simulink library "Copy_of_GFe_Lib"  (R2018b)
settings: Solver=VariableStepAuto  StartTime=0.0  StopTime=10.0  RelTol=1e-3
undefined symbols (not defined in the file or in its folder): fb, Ib2, Ki_i, Kp_i, Lf_pu, Sb, Solver_Time_Step, Time_Step, Va0, Vb0, Vb1, Vb2, Vc0, Vm0_d, Vm0_q, Vvsc0, wb, Zb
libraries: powerlib x20, Control_Lib x8, simulink x6
(part 1 of 2)
settings Model: Creator=Frederic_Colas  LastModifiedBy=Frederic_Colas
settings SFSimCC: SimUseLocalCustomCode=off
settings RTWCC: RTWUseLocalCustomCode=off

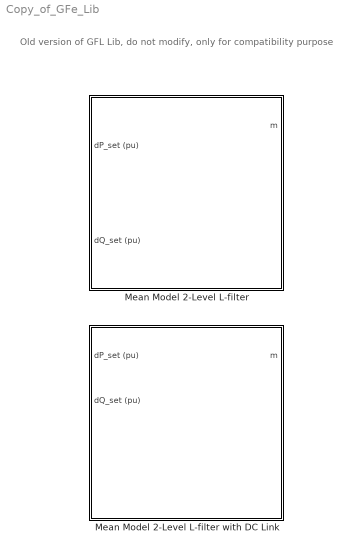
== system Copy_of_GFe_Lib ==
  note: Old version of GFL Lib, do not modify, only for compatibility purpose
  Mean Model 2-Level L-filter : Subsystem  mask(VSC){fn=50.0, Sn=1e9, Pn=1e9, Udcn=640e3, Time_Step=Time_Step, Un1=320e3, Un2=400e3, m=1, Rt_pu=0.005, Lt_pu=0.15, Lm_pu=inf, Rm_pu=inf, Tr_PLL=100, wn_i=1500, zeta_i=0.7, Kffi=on, Filtre_FF=on, w_ff=1000, QV=Reactive Power Control, w_P=10, w_V=50, w_LPF=4000, Imax=5, Iqmax=5, K_FRT=0, LFpopup=PQ, P0=0, Q0=0, V0=1.0108, Theta0=0.4912}
      mask prompts: fn "Nominal Frequency (Hz)"; Sn "Nominal Apparent Power (VA)"; Pn "Nominal Power (W)"; Udcn "Nominal DC Voltage (V)"; Time_Step "Sample Time (s)"; Un1 "VSC side Nominal Ph-Ph Voltage (V)"; Un2 "Grid side Nominal Ph-Ph Voltage (V)"; m "Transformer's ratio (p.u)"; Rt_pu "R (pu)"; Lt_pu "L (pu)"; Lm_pu "Rm (pu)"; Rm_pu "Lm (pu)"; Tr_PLL "Time response (ms)"; wn_i "Bandwidth (rad/s)"; zeta_i "Damping factor"; Kffi "Feedfoward Enable"; Filtre_FF "Filter of ff enable"; w_ff "Cutoff frequency (rad/s)"; QV "Mode"; w_P "Power control bandwidth"; w_V "Voltage control bandwidth"; w_LPF "Low-pass filters bandwidth"; Imax "Maximum current"; Iqmax "Maximum quadrature current"; K_FRT "LVRT block enabled (1) or disabled (0)"; P0 "Initial Active Power (pu)"; Q0 "Initial Reactive Power (pu)"; V0 "Initial Voltage (pu)"; Theta0 "Initial Angle (°)"
      mask init:
      | Init_Base;
      | Init_LF_L;
      | Init_GFL;
      settings: OpenFcn=|
      | NameStr = get_param(gcb,'Name');
      | open_system(gcbh, 'Mask');
      | 
      | h2AllOpenDlgs = DAStudio.ToolRoot.getOpenDialogs;
      | 
      | for i=1:length(h2AllOpenDlgs)
      |     try
      |          %disp(h2AllOpenDlgs(i).getSource.getBlock.Name);
      |         Dialog_block_name = h2AllOpenDlgs(i).getSource.getBlock.Name;
      |          %strcmp(Dialog_block_name, NameStr),
      |         if (strcmp(h2AllOpenDlgs(i).getSource.getBlock.Name, NameStr))
      |             iPos = h2AllOpenDlgs(i).position;
      |             h2AllOpenDlgs(i).position = [iPos(1)   iPos(2)   iPos(3)*1.4   iPos(4)];
      |         end
      |     end
      | end
      mask TypeOptions QV: Voltage Control | Reactive Power Control
      mask TypeOptions LFpopup: Swing | PQ | PV
      mask Callback LFpopup:
      | % Get the mask parameter values. This is a cell
      | %   array of character vectors.
      | maskStr = get_param(gcb,'LFpopup');
      | p=Simulink.Mask.get(gcb);
      | 
      | % The pop-up menu is the first mask parameter.
      | %   Check the value selected in the pop-up
      | if strcmp(maskStr,'Swing'),
      | 
      |     % Set the visibility of both parameters on when
      |     %   User-defined is selected in the pop-up.
      |     p.getParameter('P0').Visible='off';
      |     p.getParameter('Q0').Visible='off';
      |     p.getParameter('V0').Visible='on';
      |     p.getParameter('Theta0').Visible='on';
      |     set_param([gcb '/Source_For_LF'],'BusType','swing');
      | 
      | elseif strcmp(maskStr,'PQ'),
      | 
      |     % Set the visibility of both parameters on when
      |     %   User-defined is selected in the pop-up.
      |     p.getParameter('P0').Visible='on';
      |     p.getParameter('Q0').Visible='on';
      |     p.getParameter('V0').Visible='off';
      |     p.getParameter('Theta0').Visible='off';
      |     set_param([gcb '/Source_For_LF'],'BusType','PQ');
      | 
      |     % Turn off the visibility of the Value field
      |     %   when User-defined is not selected.
      | else
      | 
      |     % Set the visibility of both parameters on when
      |     %   User-defined is selected in the pop-up.
      |     p.getParameter('P0').Visible='on';
      |     p.getParameter('Q0').Visible='off';
      |     p.getParameter('V0').Visible='on';
      |     p.getParameter('Theta0').Visible='off';
      |     set_param([gcb '/Source_For_LF'],'BusType','PV');
      | 
      | end
      mask DialogControl Nominal_Param Prompt: Nominal Value
      mask DialogControl Container20 Prompt: Output Transformer
      mask DialogControl Control_Param Prompt: Control Parameter
      mask DialogControl Container13 Prompt: PLL
      mask DialogControl Container14 Prompt: Current Loop
      mask DialogControl Container11 Prompt: Outer loop
      mask DialogControl Container15 Prompt: Control gains
      mask DialogControl Container16 Prompt: Current saturations
      mask DialogControl Container21 Prompt: LVRT
      mask DialogControl LF_Param Prompt: Loadflow
      mask DialogControl Control4 Prompt: Initial Operating Point
      mask DialogControl Container24 Prompt: VSC side
      mask DialogControl LF_vsc_str Prompt: V0 = 1.0108 pu, Angle = 0.4912°
      mask DialogControl Container25 Prompt: PCC
      mask DialogControl LF_pcc_str Prompt: V0 = 1.0108 pu, Angle = 0.4912°
      mask DialogControl LF_pcc_Power_str Prompt: P0 = 0 pu, Q0 = 0 pu
      mask DialogControl UpdateLoadflow Prompt: Update Loadflow
      mask DialogControl UpdateLoadflow Callback: LoadFlow_VSC
      mask Display:
      | x1=0.05;
      | y1=0.2;
      | %
      | plot([0.5 0.5]+x1,[0.97,0.8]-y1)
      | plot([0.5 0.32]+x1,[0.80 0.71]-y1)
      | plot([0.32 0.32]+x1,[0.80 0.52]-y1)
      | plot([0.32 0.5]+x1,[0.62 0.52]-y1)
      | plot([0.5 0.5]+x1,[0.52 0.35]-y1)
      | plot([0.45 0.5 0.43]+x1,[0.59 0.52 0.51]-y1)
      | %
      | plot([0.28 0.28]+x1,[0.74 0.58]-y1)
      | plot([0.28 0.20]+x1,[0.66 0.66]-y1)
      | %
      | plot([0.5 0.63]+x1,[0.84 0.84]-y1)
      | plot([0.63 0.63]+x1,[0.84 0.72]-y1)
      | plot([0.63 0.59]+x1,[0.72 0.65]-y1)
      | plot([0.63 0.67]+x1,[0.72 0.65]-y1)
      | plot([0.59 0.67]+x1,[0.65 0.65]-y1)
      | plot([0.63 0.63]+x1,[0.65 0.47]-y1)
      | plot([0.5 0.63]+x1,[0.47 0.47]-y1)
      | plot([0.58 0.67]+x1,[0.72 0.72]-y1)
      | %
      | color('blue')
      | text(0.3,0.10,'L-Filter GFL')
      | 
      | port_label('input',1,'\DeltaP (pu)','texmode','on');
      | port_label('input',2,'\DeltaQ (pu)','texmode','on');
      | port_label('output',1,'m');
      | port_label('rconn',1,'A');
      | port_label('rconn',2,'B');
      | port_label('rconn',3,'C');
  Mean Model 2-Level L-filter with DC Link : Subsystem  mask(VSC){fn=50.0, Sn=1e9, Pn=1e9, Udcn=640e3, Time_Step=Time_Step, Un1=320e3, Un2=400e3, m=1, Rt_pu=0.005, Lt_pu=0.15, Lm_pu=inf, Rm_pu=inf, H_DC=40, Tr_PLL=100, wn_i=1500, zeta_i=0.7, Kffi=on, Filtre_FF=on, w_ff=1000, QV=Reactive Power Control, w_P=10, w_V=50, w_LPF=4000, Imax=5, Iqmax=5, K_FRT=0, LFpopup=PQ, P0=0, Q0=0, V0=1.0108, Theta0=0.4912}
      mask prompts: fn "Nominal Frequency (Hz)"; Sn "Nominal Apparent Power (VA)"; Pn "Nominal Power (W)"; Udcn "Nominal DC Voltage (V)"; Time_Step "Sample Time (s)"; Un1 "VSC side Nominal Ph-Ph Voltage (V)"; Un2 "Grid side Nominal Ph-Ph Voltage (V)"; m "Transformer's ratio (p.u)"; Rt_pu "R (pu)"; Lt_pu "L (pu)"; Lm_pu "Rm (pu)"; Rm_pu "Lm (pu)"; H_DC "DC inertias (ms)"; Tr_PLL "Time response (ms)"; wn_i "Bandwidth (rad/s)"; zeta_i "Damping factor"; Kffi "Feedfoward Enable"; Filtre_FF "Filter of ff enable"; w_ff "Cutoff frequency (rad/s)"; QV "Mode"; w_P "Power control bandwidth"; w_V "Voltage control bandwidth"; w_LPF "Low-pass filters bandwidth"; Imax "Maximum current"; Iqmax "Maximum quadrature current"; K_FRT "LVRT block enabled (1) or disabled (0)"; P0 "Initial Active Power (pu)"; Q0 "Initial Reactive Power (pu)"; V0 "Initial Voltage (pu)"; Theta0 "Initial Angle (°)"
      mask init:
      | Init_Base;
      | Init_LF_L;
      | Init_GFL;
      | Init_Cdc;
      settings: OpenFcn=|
      | NameStr = get_param(gcb,'Name');
      | open_system(gcbh, 'Mask');
      | 
      | h2AllOpenDlgs = DAStudio.ToolRoot.getOpenDialogs;
      | 
      | for i=1:length(h2AllOpenDlgs)
      |     try
      |          %disp(h2AllOpenDlgs(i).getSource.getBlock.Name);
      |         Dialog_block_name = h2AllOpenDlgs(i).getSource.getBlock.Name;
      |          %strcmp(Dialog_block_name, NameStr),
      |         if (strcmp(h2AllOpenDlgs(i).getSource.getBlock.Name, NameStr))
      |             iPos = h2AllOpenDlgs(i).position;
      |             h2AllOpenDlgs(i).position = [iPos(1)   iPos(2)   iPos(3)*1.4   iPos(4)];
      |         end
      |     end
      | end
      mask TypeOptions QV: Voltage Control | Reactive Power Control
      mask TypeOptions LFpopup: Swing | PQ | PV
      mask Callback LFpopup:
      | % Get the mask parameter values. This is a cell
      | %   array of character vectors.
      | maskStr = get_param(gcb,'LFpopup');
      | p=Simulink.Mask.get(gcb);
      | 
      | % The pop-up menu is the first mask parameter.
      | %   Check the value selected in the pop-up
      | if strcmp(maskStr,'Swing'),
      | 
      |     % Set the visibility of both parameters on when
      |     %   User-defined is selected in the pop-up.
      |     p.getParameter('P0').Visible='off';
      |     p.getParameter('Q0').Visible='off';
      |     p.getParameter('V0').Visible='on';
      |     p.getParameter('Theta0').Visible='on';
      |     set_param([gcb '/Source_For_LF'],'BusType','swing');
      | 
      | elseif strcmp(maskStr,'PQ'),
      | 
      |     % Set the visibility of both parameters on when
      |     %   User-defined is selected in the pop-up.
      |     p.getParameter('P0').Visible='on';
      |     p.getParameter('Q0').Visible='on';
      |     p.getParameter('V0').Visible='off';
      |     p.getParameter('Theta0').Visible='off';
      |     set_param([gcb '/Source_For_LF'],'BusType','PQ');
      | 
      |     % Turn off the visibility of the Value field
      |     %   when User-defined is not selected.
      | else
      | 
      |     % Set the visibility of both parameters on when
      |     %   User-defined is selected in the pop-up.
      |     p.getParameter('P0').Visible='on';
      |     p.getParameter('Q0').Visible='off';
      |     p.getParameter('V0').Visible='on';
      |     p.getParameter('Theta0').Visible='off';
      |     set_param([gcb '/Source_For_LF'],'BusType','PV');
      | 
      | end
      mask DialogControl Nominal_Param Prompt: Nominal Value
      mask DialogControl Container20 Prompt: Passive Components
      mask DialogControl Container29 Prompt: Output Transformer
      mask DialogControl Container28 Prompt: DC Link
      mask DialogControl Control_Param Prompt: Control Parameter
      mask DialogControl Container13 Prompt: PLL
      mask DialogControl Container14 Prompt: Current Loop
      mask DialogControl Container11 Prompt: Outer loop
      mask DialogControl Container15 Prompt: Control gains
      mask DialogControl Container16 Prompt: Current saturations
      mask DialogControl Container21 Prompt: LVRT
      mask DialogControl LF_Param Prompt: Loadflow
      mask DialogControl Control4 Prompt: Initial Operating Point
      mask DialogControl Container24 Prompt: VSC side
      mask DialogControl LF_vsc_str Prompt: V0 = 1.0108 pu, Angle = 0.4912°
      mask DialogControl Container25 Prompt: PCC
      mask DialogControl LF_pcc_str Prompt: V0 = 1.0108 pu, Angle = 0.4912°
      mask DialogControl LF_pcc_Power_str Prompt: P0 = 0 pu, Q0 = 0 pu
      mask DialogControl UpdateLoadflow Prompt: Update Loadflow
      mask DialogControl UpdateLoadflow Callback: LoadFlow_VSC
      mask Display:
      | x1=0.05;
      | y1=0.2;
      | %
      | plot([0.5 0.5]+x1,[0.97,0.8]-y1)
      | plot([0.5 0.32]+x1,[0.80 0.71]-y1)
      | plot([0.32 0.32]+x1,[0.80 0.52]-y1)
      | plot([0.32 0.5]+x1,[0.62 0.52]-y1)
      | plot([0.5 0.5]+x1,[0.52 0.35]-y1)
      | plot([0.45 0.5 0.43]+x1,[0.59 0.52 0.51]-y1)
      | %
      | plot([0.28 0.28]+x1,[0.74 0.58]-y1)
      | plot([0.28 0.20]+x1,[0.66 0.66]-y1)
      | %
      | plot([0.5 0.63]+x1,[0.84 0.84]-y1)
      | plot([0.63 0.63]+x1,[0.84 0.72]-y1)
      | plot([0.63 0.59]+x1,[0.72 0.65]-y1)
      | plot([0.63 0.67]+x1,[0.72 0.65]-y1)
      | plot([0.59 0.67]+x1,[0.65 0.65]-y1)
      | plot([0.63 0.63]+x1,[0.65 0.47]-y1)
      | plot([0.5 0.63]+x1,[0.47 0.47]-y1)
      | plot([0.58 0.67]+x1,[0.72 0.72]-y1)
      | %
      | color('blue')
      | text(0.3,0.10,'L-Filter GFL')
      | 
      | port_label('input',1,'\DeltaP (pu)','texmode','on');
      | port_label('input',2,'\DeltaQ (pu)','texmode','on');
      | port_label('output',1,'m');
      | port_label('rconn',1,'A');
      | port_label('rconn',2,'B');
      | port_label('rconn',3,'C');
      | port_label('lconn',1,'+');
      | port_label('lconn',2,'-');

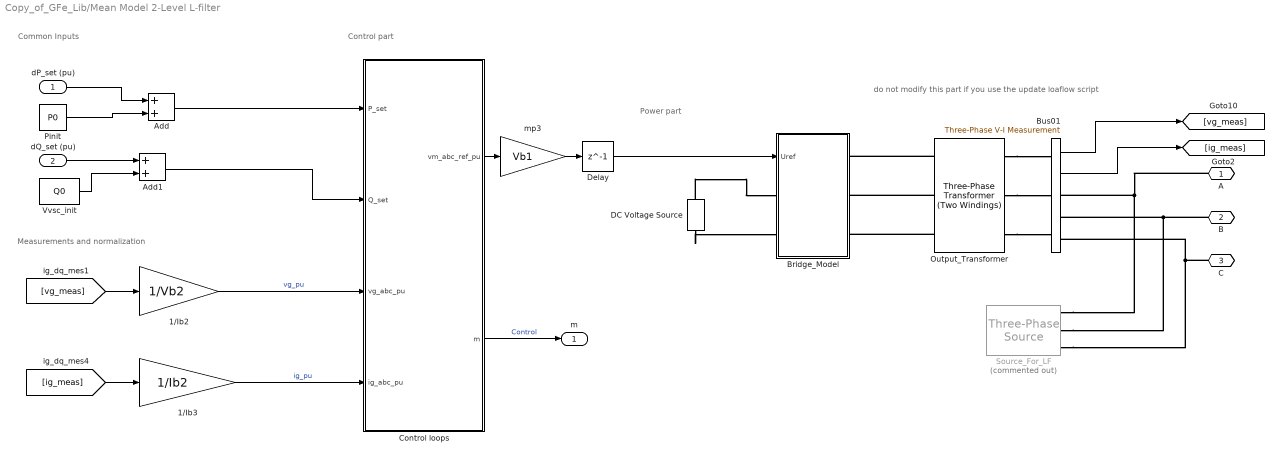
== system Copy_of_GFe_Lib/Mean Model 2-Level L-filter ==
  note: Control part
  note: Measurements and normalization
  note: Power part
  note: Common Inputs
  note: do not modify this part if you use the update loaflow script
  dP_set (pu) : Inport
  dQ_set (pu) : Inport  Port=2
  1/Ib2 : Gain  Gain=1/Vb2
  1/Ib3 : Gain  Gain=1/Ib2
  Add : Sum
  Add1 : Sum
  Bridge_Model : Subsystem
  Bus01 : powerlib/Measurements/Three-Phase V-I Measurement  VoltageMeasurement=phase-to-ground  SetLabelV=off  LabelV=Vabc  Vpu=off  VpuLL=off  CurrentMeasurement=yes  SetLabelI=off  LabelI=Iabc  Ipu=off  Pbase=100e6  Vbase=500e3  OutputType=Complex  PhasorSimulation=off  PSBequivalent=0
  Control loops : Subsystem
  DC Voltage Source : powerlib/Electrical Sources/DC Voltage Source  Amplitude=Udcn  Measurements=Voltage
  Delay : Delay  DelayLength=1  InitialCondition=[Va0 Vb0 Vc0]  SampleTime=Solver_Time_Step
  Output_Transformer : powerlib/Elements/Three-Phase Transformer (Two Windings)  Winding1Connection=Yg  Winding2Connection=Yg  CoreType=Three single-phase transformers  SetSaturation=off  Hysteresis=off  DataFile='hysteresis'  SetInitialFlux=off  Measurements=None  UNITS=pu  NominalPower=[Sn , fb]  Winding1=[Un1 , Rt_pu/2*(m^2), Lt_pu/2*(m^2)]  Winding2="[Un2*m ,  Rt_pu/2*(m^2), Lt_pu/2*(m^2)]"  Rm=Rm_pu  Lm=Lm_pu  L0=0.5  Saturation=[ 0,0 ; 0.0024,1.2 ; 1.0,1.52 ]  InitialFluxes=[ 0.8 , -0.8 , 0.7 ]  BreakLoop=off  DiscreteSolver=Trapezoidal iterative  DataType=off  TransfoNumber=1
  Pinit : Constant  Value=P0
  Source_For_LF : powerlib/Electrical Sources/Three-Phase Source  Commented=on  InternalConnection=Yg  VoltagePhases=off  Voltage=(400000)*1.01081  PhaseAngle=0.4912  Voltage_phases=[25e3 25e3 25e3]/sqrt(3)  PhaseAngles_phases=[0 -120 +120]  Frequency=fb  NonIdealSource=off  SpecifyImpedance=off  Resistance=0  Inductance=0  ShortCircuitLevel=100e6  BaseVoltage=Un  XRratio=7  BusType=PQ  Pref=P0*Sb  Qref=Q0*Sb  Prefabc=[10e3, 10e3, 10e3]  Qrefabc=[0, 0, 0]  Qmin=-inf  Qmax=inf
  Vvsc_init : Constant  Value=Q0
  mp3 : Gain  Gain=Vb1
  A : PMIOPort  Side=Right
  B : PMIOPort  Port=2  Side=Right
  C : PMIOPort  Port=3  Side=Right
  m : Outport  VectorParamsAs1DForOutWhenUnconnected=off
  wires:
  [ig_meas] -> 1/Ib3/1
  dQ_set (pu)/1 -> Add1/1
  Vvsc_init/1 -> Add1/2
  Pinit/1 -> Add/2
  dP_set (pu)/1 -> Add/1
  Add1/1 -> Control loops/2(Q_set)
  Control loops/1(vm_abc_ref_pu) -> mp3/1
  [vg_meas] -> 1/Ib2/1
  1/Ib2/1 -> Control loops/3(vg_abc_pu)  "vg_pu"
  1/Ib3/1 -> Control loops/4(ig_abc_pu)  "ig_pu"
  mp3/1 -> Delay/1
  Control loops/2(m) -> m/1  "Control"
  Add/1 -> Control loops/1(P_set)
  Bus01/1 -> [vg_meas]
  Delay/1 -> Bridge_Model/1(Uref)
  Bus01/2 -> [ig_meas]
  connections:
  B/RConn1 -- Source_For_LF/RConn2 -- Bus01/RConn2
  C/RConn1 -- Source_For_LF/RConn3 -- Bus01/RConn3
  A/RConn1 -- Source_For_LF/RConn1 -- Bus01/RConn1
  DC Voltage Source/RConn1 -- Bridge_Model/LConn1
  Output_Transformer/LConn3 -- Bridge_Model/RConn3
  Output_Transformer/LConn1 -- Bridge_Model/RConn1
  DC Voltage Source/LConn1 -- Bridge_Model/LConn2
  Output_Transformer/RConn2 -- Bus01/LConn2
  Output_Transformer/RConn1 -- Bus01/LConn1
  Output_Transformer/LConn2 -- Bridge_Model/RConn2
  Output_Transformer/RConn3 -- Bus01/LConn3

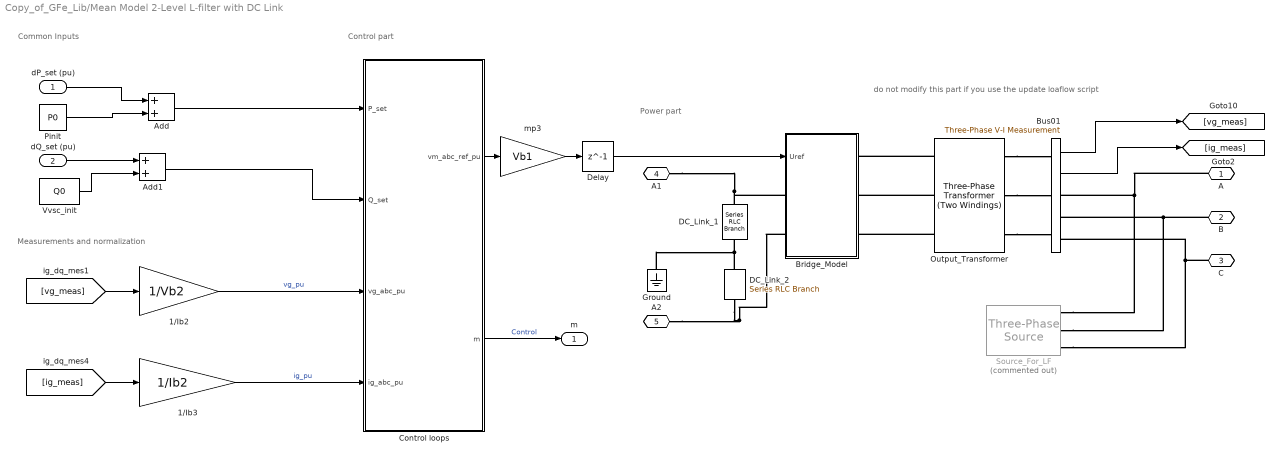
== system Copy_of_GFe_Lib/Mean Model 2-Level L-filter with DC Link ==
  note: Control part
  note: Measurements and normalization
  note: Power part
  note: Common Inputs
  note: do not modify this part if you use the update loaflow script
  dP_set (pu) : Inport
  dQ_set (pu) : Inport  Port=2
  1/Ib2 : Gain  Gain=1/Vb2
  1/Ib3 : Gain  Gain=1/Ib2
  Add : Sum
  Add1 : Sum
  Bridge_Model : Subsystem
  Bus01 : powerlib/Measurements/Three-Phase V-I Measurement  VoltageMeasurement=phase-to-ground  SetLabelV=off  LabelV=Vabc  Vpu=off  VpuLL=off  CurrentMeasurement=yes  SetLabelI=off  LabelI=Iabc  Ipu=off  Pbase=100e6  Vbase=500e3  OutputType=Complex  PhasorSimulation=off  PSBequivalent=0
  Control loops : Subsystem
  DC_Link_1 : powerlib/Elements/Series RLC Branch  LConnTagsString=__new0  RConnTagsString=__new0  BranchType=C  Resistance=1  Inductance=1e-3  SetiL0=off  InitialCurrent=0  Capacitance=0.00039063  Setx0=on  InitialVoltage=Udcn/2  Measurements=None
  DC_Link_2 : powerlib/Elements/Series RLC Branch  LConnTagsString=__new0  RConnTagsString=__new0  BranchType=C  Resistance=1  Inductance=1e-3  SetiL0=off  InitialCurrent=0  Capacitance=0.00039063  Setx0=on  InitialVoltage=Udcn/2  Measurements=None
  Delay : Delay  DelayLength=1  InitialCondition=[Va0 Vb0 Vc0]  SampleTime=Solver_Time_Step
  Ground : powerlib/Elements/Ground  LConnTagsString=a
  Output_Transformer : powerlib/Elements/Three-Phase Transformer (Two Windings)  Winding1Connection=Yg  Winding2Connection=Yg  CoreType=Three single-phase transformers  SetSaturation=off  Hysteresis=off  DataFile='hysteresis'  SetInitialFlux=off  Measurements=None  UNITS=pu  NominalPower=[Sn , fb]  Winding1=[Un1 , Rt_pu/2*(m^2), Lt_pu/2*(m^2)]  Winding2="[Un2*m ,  Rt_pu/2*(m^2), Lt_pu/2*(m^2)]"  Rm=Rm_pu  Lm=Lm_pu  L0=0.5  Saturation=[ 0,0 ; 0.0024,1.2 ; 1.0,1.52 ]  InitialFluxes=[ 0.8 , -0.8 , 0.7 ]  BreakLoop=off  DiscreteSolver=Trapezoidal iterative  DataType=off  TransfoNumber=1
  Pinit : Constant  Value=P0
  Source_For_LF : powerlib/Electrical Sources/Three-Phase Source  Commented=on  InternalConnection=Yg  VoltagePhases=off  Voltage=(400000)*1.01081  PhaseAngle=0.4912  Voltage_phases=[25e3 25e3 25e3]/sqrt(3)  PhaseAngles_phases=[0 -120 +120]  Frequency=fb  NonIdealSource=off  SpecifyImpedance=off  Resistance=0  Inductance=0  ShortCircuitLevel=100e6  BaseVoltage=Un  XRratio=7  BusType=PQ  Pref=P0*Sb  Qref=Q0*Sb  Prefabc=[10e3, 10e3, 10e3]  Qrefabc=[0, 0, 0]  Qmin=-inf  Qmax=inf
  Vvsc_init : Constant  Value=Q0
  mp3 : Gain  Gain=Vb1
  A : PMIOPort  Side=Right
  B : PMIOPort  Port=2  Side=Right
  C : PMIOPort  Port=3  Side=Right
  A1 : PMIOPort  Port=4  Side=Left
  A2 : PMIOPort  Port=5  Side=Left
  m : Outport  VectorParamsAs1DForOutWhenUnconnected=off
  wires:
  [ig_meas] -> 1/Ib3/1
  dQ_set (pu)/1 -> Add1/1
  Vvsc_init/1 -> Add1/2
  Pinit/1 -> Add/2
  dP_set (pu)/1 -> Add/1
  Add1/1 -> Control loops/2(Q_set)
  Control loops/1(vm_abc_ref_pu) -> mp3/1
  [vg_meas] -> 1/Ib2/1
  1/Ib2/1 -> Control loops/3(vg_abc_pu)  "vg_pu"
  1/Ib3/1 -> Control loops/4(ig_abc_pu)  "ig_pu"
  mp3/1 -> Delay/1
  Control loops/2(m) -> m/1  "Control"
  Add/1 -> Control loops/1(P_set)
  Bus01/1 -> [vg_meas]
  Delay/1 -> Bridge_Model/1(Uref)
  Bus01/2 -> [ig_meas]
  connections:
  B/RConn1 -- Source_For_LF/RConn2 -- Bus01/RConn2
  C/RConn1 -- Source_For_LF/RConn3 -- Bus01/RConn3
  A/RConn1 -- Source_For_LF/RConn1 -- Bus01/RConn1
  Output_Transformer/LConn3 -- Bridge_Model/RConn3
  Output_Transformer/LConn1 -- Bridge_Model/RConn1
  Output_Transformer/RConn2 -- Bus01/LConn2
  Output_Transformer/RConn1 -- Bus01/LConn1
  Output_Transformer/LConn2 -- Bridge_Model/RConn2
  Output_Transformer/RConn3 -- Bus01/LConn3
  DC_Link_1/LConn1 -- A1/RConn1 -- Bridge_Model/LConn1
  DC_Link_2/RConn1 -- Bridge_Model/LConn2 -- A2/RConn1
  DC_Link_1/RConn1 -- DC_Link_2/LConn1 -- Ground/LConn1

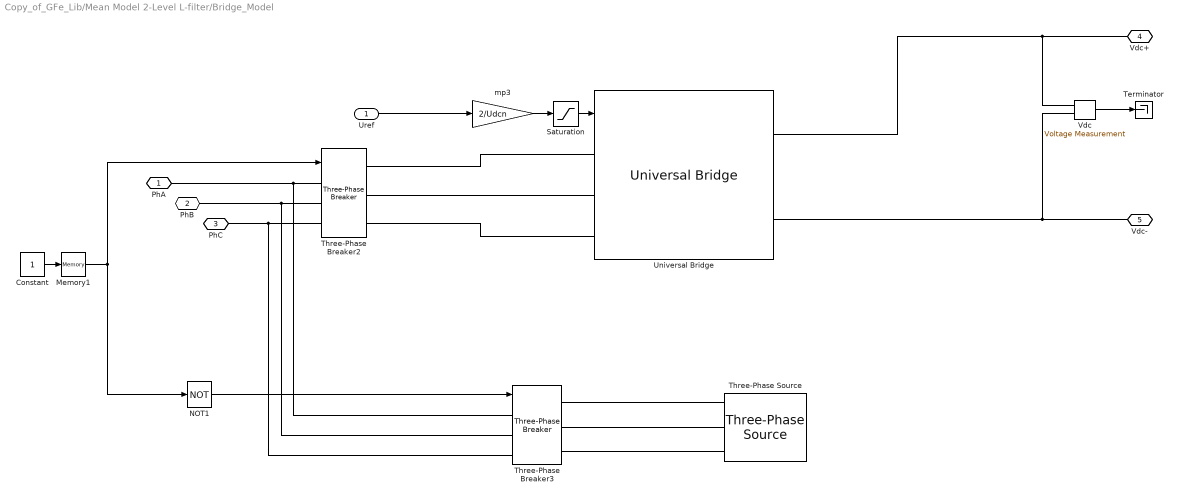
== system Copy_of_GFe_Lib/Mean Model 2-Level L-filter/Bridge_Model ==
  Uref : Inport
  Constant : Constant
  Memory1 : Memory
  NOT1 : Logic  Operator=NOT  IconShape=distinctive  AllPortsSameDT=off  OutDataTypeStr=boolean
  Saturation : Saturate  UpperLimit=1  LowerLimit=-1
  Terminator : Terminator
  Three-Phase Breaker2 : powerlib/Elements/Three-Phase Breaker  InitialState=open  SwitchA=on  SwitchB=on  SwitchC=on  SwitchTimes="[4/60  10/60]"  External=on  BreakerResistance=1e-5*Zb  SnubberResistance=1e6  SnubberCapacitance=inf  Measurements=None
  Three-Phase Breaker3 : powerlib/Elements/Three-Phase Breaker  InitialState=closed  SwitchA=on  SwitchB=on  SwitchC=on  SwitchTimes="[4/60  10/60]"  External=on  BreakerResistance=1e-5*Zb  SnubberResistance=1e6  SnubberCapacitance=inf  Measurements=None
  Three-Phase Source : powerlib/Electrical Sources/Three-Phase Source  InternalConnection=Yg  VoltagePhases=off  Voltage=Vvsc0*Un1  PhaseAngle=Theta_vsc0  Voltage_phases=[25e3 25e3 25e3]/sqrt(3)  PhaseAngles_phases=[0 -120 +120]  Frequency=fb  NonIdealSource=off  SpecifyImpedance=off  Resistance=0  Inductance=0  ShortCircuitLevel=100e6  BaseVoltage=VSC01_Un1  XRratio=7  BusType=swing  Pref=0.3  Qref=0  Prefabc=[10e3, 10e3, 10e3]  Qrefabc=[0, 0, 0]  Qmin=-Inf  Qmax=Inf
  Universal Bridge : powerlib/Power Electronics/Universal Bridge  Arms=3  SnubberResistance=1e5  SnubberCapacitance=inf  Device=Average-model based VSC  Ron=1e-3  Lon=0  ForwardVoltages="[  0  0  ]"  ForwardVoltage=0  GTOparameters=[ 10e-6 , 20e-6 ]  IGBTparameters=[ 1e-6 , 2e-6 ]  Measurements=None  Measurements_2=None  converterType=Rectifier
  Vdc : powerlib/Measurements/Voltage Measurement  PhasorSimulation=off  OutputType=Complex  PSBequivalent=0
  mp3 : Gain  Gain=2/Udcn
  PhA : PMIOPort  Side=Right
  PhB : PMIOPort  Port=2  Side=Right
  PhC : PMIOPort  Port=3  Side=Right
  Vdc+ : PMIOPort  Port=4  Side=Left
  Vdc- : PMIOPort  Port=5  Side=Left
  wires:
  Vdc/1 -> Terminator/1
  Uref/1 -> mp3/1
  mp3/1 -> Saturation/1
  Constant/1 -> Memory1/1
  NOT1/1 -> Three-Phase Breaker3/1
  Saturation/1 -> Universal Bridge/1
  Memory1/1 -> Three-Phase Breaker2/1, NOT1/1
  connections:
  Vdc-/RConn1 -- Universal Bridge/RConn2 -- Vdc/LConn2
  Vdc+/RConn1 -- Universal Bridge/RConn1 -- Vdc/LConn1
  PhC/RConn1 -- Three-Phase Breaker3/LConn3 -- Three-Phase Breaker2/LConn3
  PhB/RConn1 -- Three-Phase Breaker3/LConn2 -- Three-Phase Breaker2/LConn2
  PhA/RConn1 -- Three-Phase Breaker3/LConn1 -- Three-Phase Breaker2/LConn1
  Three-Phase Breaker2/RConn3 -- Universal Bridge/LConn3
  Three-Phase Breaker2/RConn2 -- Universal Bridge/LConn2
  Three-Phase Breaker2/RConn1 -- Universal Bridge/LConn1
  Three-Phase Breaker3/RConn1 -- Three-Phase Source/RConn1
  Three-Phase Breaker3/RConn2 -- Three-Phase Source/RConn2
  Three-Phase Breaker3/RConn3 -- Three-Phase Source/RConn3

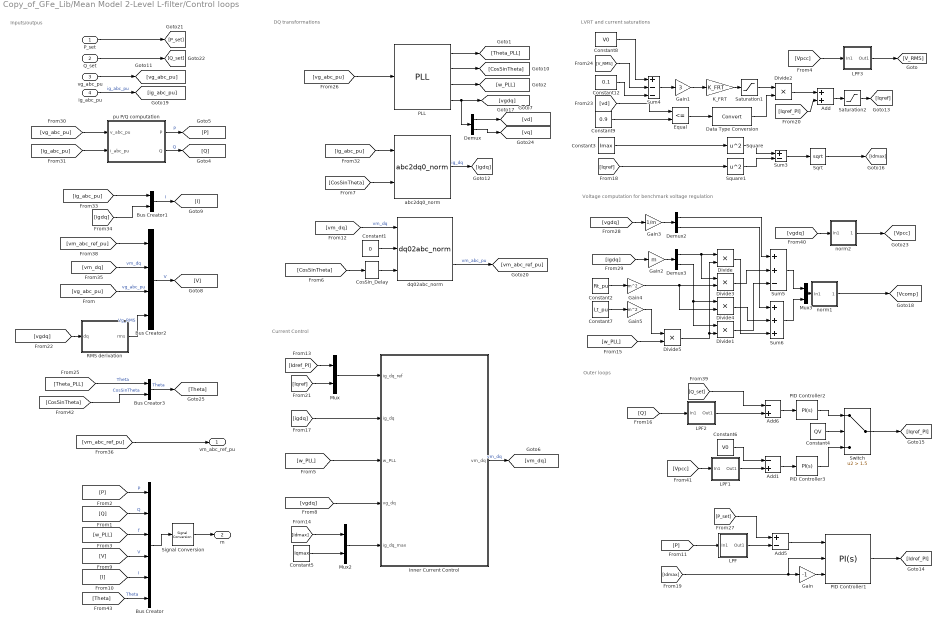
== system Copy_of_GFe_Lib/Mean Model 2-Level L-filter/Control loops ==
  note: Voltage computation for benchmark voltage regulation
  note: LVRT and current saturations
  note: Outer loops
  note: Current Control
  note: DQ transformations
  note: Inputs/outpus
  P_set : Inport
  Q_set : Inport  Port=2
  vg_abc_pu : Inport  Port=3
  ig_abc_pu : Inport  Port=4
  " pu P/Q computation" : Subsystem  DialogController=POWERSYS.PowerSysDialog
  Add : Sum
  Add1 : Sum  Inputs=-+
  Add5 : Sum  Inputs=+-
  Add6 : Sum  Inputs=-+
  Bus Creator : BusCreator  Inputs=6
  Bus Creator1 : BusCreator  Inputs=2
  Bus Creator2 : BusCreator  Inputs=4
  Bus Creator3 : BusCreator  Inputs=2
  Constant1 : Constant  Value=0
  Constant12 : Constant  Value=0.1
  Constant2 : Constant  Value=Rt_pu
  Constant3 : Constant  Value=Imax
  Constant4 : Constant  Value=QV
  Constant5 : Constant  Value=Iqmax
  Constant6 : Constant  Value=V0
  Constant7 : Constant  Value=Lt_pu
  Constant8 : Constant  Value=V0
  Constant9 : Constant  Value=0.9
  CosSin_Delay : Control_Lib/CosSin_Delay  dTheta=wb*Solver_Time_Step
      settings: SourceProductName=VSC4SPS
  Data Type Conversion : DataTypeConversion
  Demux : Demux  Outputs=[1 1]
  Demux2 : Demux  Outputs=2
  Demux3 : Demux  Outputs=2
  Divide{,1..5} (6 alike) : Product  Inputs=**
  Equal : RelationalOperator  Operator=<=  OutDataTypeStr=boolean  RndMeth=Simplest
  Gain : Gain  Gain=-1
  Gain1 : Gain  Gain=3
  Gain2 : Gain  Gain=m
  Gain3 : Gain  Gain=1/m
  Gain4 : Gain  Gain=m^2
  Gain5 : Gain  Gain=m^2
  Inner Current Control : Subsystem
  K_FRT : Gain  Gain=K_FRT
  LPF : Subsystem
  LPF1 : Subsystem
  LPF2 : Subsystem
  LPF3 : Subsystem
  Mux : Mux  Inputs=2
  Mux2 : Mux  Inputs=2
  Mux3 : Mux  Inputs=2
  PID Controller1 : simulink/Continuous/PID Controller  Controller=PI  Form=Parallel  TimeDomain=Continuous-time  SampleTime=-1  IntegratorMethod=Forward Euler  FilterMethod=Forward Euler  ControllerParametersSource=internal  P=w_P/w_LPF  I=w_P  D=0  UseFilter=on  N=100  TunerSelectOption=Transfer Function Based (PID Tuner App)  InitialConditionSource=internal  InitialConditionForIntegrator=P0/V0  InitialConditionForFilter=0  DifferentiatorICPrevScaledInput=0  ExternalReset=none  TrackingMode=off  Kt=1  LimitOutput=on  UpperSaturationLimit=inf  LowerSaturationLimit=-inf  LinearizeAsGain=on  AntiWindupMode=clamping  Kb=1  POutMin=[]  POutMax=[]  IOutMin=[]  IOutMax=[]  DOutMin=[]  DOutMax=[]  NOutMin=[]  NOutMax=[]  SumOutMin=[]  SumOutMax=[]  SaturationOutMin=[]  SaturationOutMax=[]  PParamMin=[]  PParamMax=[]  IParamMin=[]  IParamMax=[]  DParamMin=[]  DParamMax=[]  NParamMin=[]  NParamMax=[]  KbParamMin=[]  KbParamMax=[]  KtParamMin=[]  KtParamMax=[]  KbOutMin=[]  KbOutMax=[]  KtOutMin=[]  KtOutMax=[]  IntegratorOutMin=[]  IntegratorOutMax=[]  FilterOutMin=[]  FilterOutMax=[]  SumI1OutMin=[]  SumI1OutMax=[]  SumI2OutMin=[]  SumI2OutMax=[]  SumI3OutMin=[]  SumI3OutMax=[]  SumI4OutMin=[]  SumI4OutMax=[]  SumDOutMin=[]  SumDOutMax=[]  DifferentiatorOutMin=[]  DifferentiatorOutMax=[]  FilterDiffOutCoefMin=[]  FilterDiffOutCoefMax=[]  ReciprocalOutMin=[]  ReciprocalOutMax=[]  SumDenOutMin=[]  SumDenOutMax=[]  SumNumOutMin=[]  SumNumOutMax=[]  DivideOutMin=[]  DivideOutMax=[]  IntegratorContinuousStateAttributes=''  IntegratorStateMustResolveToSignalObject=off  IntegratorRTWStateStorageClass=Auto  FilterContinuousStateAttributes=''  FilterStateMustResolveToSignalObject=off  FilterRTWStateStorageClass=Auto  ParallelPVariant=InternalParameters  IdealPVariant=Disabled  IVariant=InternalParameters  DVariant=Disabled  IntegratorVariant=Continuous  SatVariant=External  AWVariant=ContClampingParallel  PCopyVariant=Disabled  TRVariant=Disabled  FdbkBlocksVariant=Forward  IdealPFdbkVariant=Disabled  SatFdbkVariant=Disabled  DerivativeFilterVariant=Disabled  NVariant=Disabled  NCopyVariant=Disabled_SignalSpec  FilterICVariant=Disabled  IntegratorICVariant=InternalICs  ExternalResetVariant=Disabled  TRSumVariant=Passthrough  SumFdbkVariant=Disabled  SumVariant=Sum_PI
  PID Controller2 : simulink/Continuous/PID Controller  Controller=PI  Form=Parallel  TimeDomain=Continuous-time  SampleTime=-1  IntegratorMethod=Forward Euler  FilterMethod=Forward Euler  ControllerParametersSource=internal  P=w_P/w_LPF  I=w_P  D=0  UseFilter=on  N=100  TunerSelectOption=Transfer Function Based (PID Tuner App)  InitialConditionSource=internal  InitialConditionForIntegrator=-Q0/V0  InitialConditionForFilter=0  DifferentiatorICPrevScaledInput=0  ExternalReset=none  TrackingMode=off  Kt=1  LimitOutput=on  UpperSaturationLimit=Iqmax  LowerSaturationLimit=-Iqmax  LinearizeAsGain=on  AntiWindupMode=clamping  Kb=1  POutMin=[]  POutMax=[]  IOutMin=[]  IOutMax=[]  DOutMin=[]  DOutMax=[]  NOutMin=[]  NOutMax=[]  SumOutMin=[]  SumOutMax=[]  SaturationOutMin=[]  SaturationOutMax=[]  PParamMin=[]  PParamMax=[]  IParamMin=[]  IParamMax=[]  DParamMin=[]  DParamMax=[]  NParamMin=[]  NParamMax=[]  KbParamMin=[]  KbParamMax=[]  KtParamMin=[]  KtParamMax=[]  KbOutMin=[]  KbOutMax=[]  KtOutMin=[]  KtOutMax=[]  IntegratorOutMin=[]  IntegratorOutMax=[]  FilterOutMin=[]  FilterOutMax=[]  SumI1OutMin=[]  SumI1OutMax=[]  SumI2OutMin=[]  SumI2OutMax=[]  SumI3OutMin=[]  SumI3OutMax=[]  SumI4OutMin=[]  SumI4OutMax=[]  SumDOutMin=[]  SumDOutMax=[]  DifferentiatorOutMin=[]  DifferentiatorOutMax=[]  FilterDiffOutCoefMin=[]  FilterDiffOutCoefMax=[]  ReciprocalOutMin=[]  ReciprocalOutMax=[]  SumDenOutMin=[]  SumDenOutMax=[]  SumNumOutMin=[]  SumNumOutMax=[]  DivideOutMin=[]  DivideOutMax=[]  IntegratorContinuousStateAttributes=''  IntegratorStateMustResolveToSignalObject=off  IntegratorRTWStateStorageClass=Auto  FilterContinuousStateAttributes=''  FilterStateMustResolveToSignalObject=off  FilterRTWStateStorageClass=Auto  ParallelPVariant=InternalParameters  IdealPVariant=Disabled  IVariant=InternalParameters  DVariant=Disabled  IntegratorVariant=Continuous  SatVariant=Enabled  AWVariant=ContClampingParallel  PCopyVariant=Disabled  TRVariant=Disabled  FdbkBlocksVariant=Forward  IdealPFdbkVariant=Disabled  SatFdbkVariant=Disabled  DerivativeFilterVariant=Disabled  NVariant=Disabled  NCopyVariant=Disabled_SignalSpec  FilterICVariant=Disabled  IntegratorICVariant=InternalICs  ExternalResetVariant=Disabled  TRSumVariant=Passthrough  SumFdbkVariant=Disabled  SumVariant=Sum_PI
  PID Controller3 : simulink/Continuous/PID Controller  Controller=PI  Form=Parallel  TimeDomain=Continuous-time  SampleTime=-1  IntegratorMethod=Forward Euler  FilterMethod=Forward Euler  ControllerParametersSource=internal  P=w_V/w_LPF  I=w_V  D=0  UseFilter=on  N=100  TunerSelectOption=Transfer Function Based (PID Tuner App)  InitialConditionSource=internal  InitialConditionForIntegrator=-Q0/V0  InitialConditionForFilter=0  DifferentiatorICPrevScaledInput=0  ExternalReset=none  TrackingMode=off  Kt=1  LimitOutput=on  UpperSaturationLimit=Iqmax  LowerSaturationLimit=-Iqmax  LinearizeAsGain=on  AntiWindupMode=clamping  Kb=1  POutMin=[]  POutMax=[]  IOutMin=[]  IOutMax=[]  DOutMin=[]  DOutMax=[]  NOutMin=[]  NOutMax=[]  SumOutMin=[]  SumOutMax=[]  SaturationOutMin=[]  SaturationOutMax=[]  PParamMin=[]  PParamMax=[]  IParamMin=[]  IParamMax=[]  DParamMin=[]  DParamMax=[]  NParamMin=[]  NParamMax=[]  KbParamMin=[]  KbParamMax=[]  KtParamMin=[]  KtParamMax=[]  KbOutMin=[]  KbOutMax=[]  KtOutMin=[]  KtOutMax=[]  IntegratorOutMin=[]  IntegratorOutMax=[]  FilterOutMin=[]  FilterOutMax=[]  SumI1OutMin=[]  SumI1OutMax=[]  SumI2OutMin=[]  SumI2OutMax=[]  SumI3OutMin=[]  SumI3OutMax=[]  SumI4OutMin=[]  SumI4OutMax=[]  SumDOutMin=[]  SumDOutMax=[]  DifferentiatorOutMin=[]  DifferentiatorOutMax=[]  FilterDiffOutCoefMin=[]  FilterDiffOutCoefMax=[]  ReciprocalOutMin=[]  ReciprocalOutMax=[]  SumDenOutMin=[]  SumDenOutMax=[]  SumNumOutMin=[]  SumNumOutMax=[]  DivideOutMin=[]  DivideOutMax=[]  IntegratorContinuousStateAttributes=''  IntegratorStateMustResolveToSignalObject=off  IntegratorRTWStateStorageClass=Auto  FilterContinuousStateAttributes=''  FilterStateMustResolveToSignalObject=off  FilterRTWStateStorageClass=Auto  ParallelPVariant=InternalParameters  IdealPVariant=Disabled  IVariant=InternalParameters  DVariant=Disabled  IntegratorVariant=Continuous  SatVariant=Enabled  AWVariant=ContClampingParallel  PCopyVariant=Disabled  TRVariant=Disabled  FdbkBlocksVariant=Forward  IdealPFdbkVariant=Disabled  SatFdbkVariant=Disabled  DerivativeFilterVariant=Disabled  NVariant=Disabled  NCopyVariant=Disabled_SignalSpec  FilterICVariant=Disabled  IntegratorICVariant=InternalICs  ExternalResetVariant=Disabled  TRSumVariant=Passthrough  SumFdbkVariant=Disabled  SumVariant=Sum_PI
  PLL : Control_Lib/PLL  fb=fb  wn_PLL=wn_PLL  zeta_PLL=zeta_PLL  Theta0=Theta0
      settings: SourceProductName=VSC4SPS
  RMS derivation : Subsystem
  Saturation1 : Saturate  UpperLimit=Imax  LowerLimit=-Imax
  Saturation2 : Saturate  UpperLimit=Imax  LowerLimit=-Imax
  Signal Conversion : SignalConversion  OverrideOpt=off
  Sqrt : Sqrt  SaturateOnIntegerOverflow=on
  Square : Math  Operator=square  SaturateOnIntegerOverflow=on
  Square1 : Math  Operator=square  SaturateOnIntegerOverflow=on
  Sum3 : Sum  Inputs=+-
  Sum4 : Sum  Inputs=+--
  Sum5 : Sum  Inputs=++-
  Sum6 : Sum  Inputs=+++
  Switch : Switch  Criteria=u2 > Threshold  Threshold=1.5
  abc2dq0_norm : Control_Lib/abc2dq0_norm  referenceAxisMode=Reference axis at 90 degrees behind phase_a  baseUpdateGain=1/sqrt(3)
      settings: SourceProductName=VSC4SPS
  dq02abc_norm : Control_Lib/dq02abc_norm  referenceAxisMode=Reference axis at 90 degrees behind phase_a  baseUpdateGain=sqrt(3)
      settings: SourceProductName=VSC4SPS
  norm1 : Subsystem
  norm2 : Subsystem
  vm_abc_ref_pu : Outport  VectorParamsAs1DForOutWhenUnconnected=off
  m : Outport  Port=2  VectorParamsAs1DForOutWhenUnconnected=off
  wires:
  [vg_abc_pu] -> Bus Creator2/3  "vg_abc_pu"
  Constant1/1 -> dq02abc_norm/2
  Mux/1 -> Inner Current Control/1(ig_dq_ref)
  Signal Conversion/1 -> m/1
  [P] -> Bus Creator/1  "P"
  [Q] -> Bus Creator/2  "Q"
  [w_PLL] -> Bus Creator/3  "f"
  dq02abc_norm/2 -> [vm_abc_ref_pu]  "vm_abc_pu"
  " pu P/Q computation"/2(Q) -> [Q]  "Q"
  [vm_dq] -> dq02abc_norm/1  "vm_dq"
  [w_PLL] -> Inner Current Control/3(w_PLL)
  Inner Current Control/1(vm_dq) -> [vm_dq]  "vm_dq"
  vg_abc_pu/1 -> [vg_abc_pu]
  " pu P/Q computation"/1(P) -> [P]  "P"
  ig_abc_pu/1 -> [ig_abc_pu]  "ig_abc_pu"
  abc2dq0_norm/2 -> [igdq]  "ig_dq"
  [CosSinTheta] -> CosSin_Delay/1
  [CosSinTheta] -> abc2dq0_norm/2
  Bus Creator2/1 -> [V]  "V"
  [V] -> Bus Creator/4  "V"
  Bus Creator/1 -> Signal Conversion/1
  Bus Creator1/1 -> [I]  "I"
  [I] -> Bus Creator/5  "I"
  LPF2/1(Out1) -> Add6/2
  P_set/1 -> [P_set]
  Add6/1 -> PID Controller2/1
  [P] -> LPF/1(In1)
  Add5/1 -> PID Controller1/1
  [Iqref] -> Mux/2
  [Idref_PI] -> Mux/1
  [igdq] -> Inner Current Control/2(ig_dq)
  Saturation2/1 -> [Iqref]
  Sum4/1 -> Gain1/1
  [V_RMS] -> Sum4/2
  K_FRT/1 -> Saturation1/1
  Saturation1/1 -> Divide2/1
  Equal/1 -> Data Type Conversion/1
  Data Type Conversion/1 -> Divide2/2
  [vd] -> Equal/1
  Divide2/1 -> Add/1
  Constant12/1 -> Sum4/3
  Constant8/1 -> Sum4/1
  Constant9/1 -> Equal/2
  Constant4/1 -> Switch/2
  Add/1 -> Saturation2/1
  [Iqref_PI] -> Add/2
  Mux2/1 -> Inner Current Control/5(ig_dq_max)
  Constant5/1 -> Mux2/2
  [Idmax] -> Mux2/1
  [Q] -> LPF2/1(In1)
  Q_set/1 -> [Q_set]
  PID Controller2/1 -> Switch/1
  Add1/1 -> PID Controller3/1
  LPF1/1(Out1) -> Add1/2
  PID Controller3/1 -> Switch/3
  Square1/1 -> Sum3/2
  Sqrt/1 -> [Idmax]
  Sum3/1 -> Sqrt/1
  Constant3/1 -> Square/1
  Square/1 -> Sum3/1
  [Iqref] -> Square1/1
  Gain/1 -> PID Controller1/3
  [Idmax] -> PID Controller1/2, Gain/1
  Gain1/1 -> K_FRT/1
  Sum5/1 -> Mux3/1
  [vgdq] -> Gain3/1
  Demux2/2 -> Sum6/1
  Gain3/1 -> Demux2/1
  Constant2/1 -> Gain4/1
  norm1/1(Out1) -> [Vcomp]
  Divide1/1 -> Sum5/3
  Sum6/1 -> Mux3/2
  Mux3/1 -> norm1/1(In1)
  Divide/1 -> Sum6/3
  Divide5/1 -> Divide/2, Divide1/2
  Demux2/1 -> Sum5/1
  Divide3/1 -> Sum5/2
  Demux3/2 -> Divide1/1, Divide4/1
  Divide4/1 -> Sum6/2
  Demux3/1 -> Divide/1, Divide3/1
  PLL/1 -> [Theta_PLL]
  PLL/2 -> [CosSinTheta]
  PLL/3 -> [w_PLL]
  [w_PLL] -> Divide5/2
  Constant7/1 -> Gain5/1
  [Vpcc] -> LPF1/1(In1)
  Constant6/1 -> Add1/1
  [vg_abc_pu] -> PLL/1
  [vg_abc_pu] -> " pu P/Q computation"/1(v_abc_pu)
  [ig_abc_pu] -> " pu P/Q computation"/2(i_abc_pu)
  [ig_abc_pu] -> abc2dq0_norm/1
  [ig_abc_pu] -> Bus Creator1/1
  [igdq] -> Bus Creator1/2
  [vm_dq] -> Bus Creator2/2  "vm_dq"
  [vm_abc_ref_pu] -> vm_abc_ref_pu/1
  [vm_abc_ref_pu] -> Bus Creator2/1
  [vgdq] -> Inner Current Control/4(vg_dq)
  [P_set] -> Add5/1
  [Q_set] -> Add6/1
  [igdq] -> Gain2/1
  Gain2/1 -> Demux3/1
  Gain5/1 -> Divide5/1
  Gain4/1 -> Divide4/2, Divide3/2
  [vgdq] -> norm2/1(In1)
  norm2/1(Out1) -> [Vpcc]
  PLL/4 -> Demux/1, [vgdq]
  Demux/1 -> [vd]
  Demux/2 -> [vq]
  PID Controller1/1 -> [Idref_PI]
  Switch/1 -> [Iqref_PI]
  LPF/1(Out1) -> Add5/2
  [vgdq] -> RMS derivation/1(dq)
  RMS derivation/1(rms) -> Bus Creator2/4  "Vg_RMS"
  [Theta_PLL] -> Bus Creator3/1  "Theta"
  [CosSinTheta] -> Bus Creator3/2  "CosSinTheta"
  Bus Creator3/1 -> [Theta]  "Theta"
  [Theta] -> Bus Creator/6  "Theta"
  CosSin_Delay/1 -> dq02abc_norm/3
  LPF3/1(Out1) -> [V_RMS]
  [Vpcc] -> LPF3/1(In1)

== system Copy_of_GFe_Lib/Mean Model 2-Level L-filter with DC Link/Bridge_Model ==
  Uref : Inport
  Constant : Constant
  Memory1 : Memory
  NOT1 : Logic  Operator=NOT  IconShape=distinctive  AllPortsSameDT=off  OutDataTypeStr=boolean
  Saturation : Saturate  UpperLimit=1  LowerLimit=-1
  Terminator : Terminator
  Three-Phase Breaker2 : powerlib/Elements/Three-Phase Breaker  InitialState=open  SwitchA=on  SwitchB=on  SwitchC=on  SwitchTimes="[4/60  10/60]"  External=on  BreakerResistance=1e-5*Zb  SnubberResistance=1e6  SnubberCapacitance=inf  Measurements=None
  Three-Phase Breaker3 : powerlib/Elements/Three-Phase Breaker  InitialState=closed  SwitchA=on  SwitchB=on  SwitchC=on  SwitchTimes="[4/60  10/60]"  External=on  BreakerResistance=1e-5*Zb  SnubberResistance=1e6  SnubberCapacitance=inf  Measurements=None
  Three-Phase Source : powerlib/Electrical Sources/Three-Phase Source  InternalConnection=Yg  VoltagePhases=off  Voltage=Vvsc0*Un1  PhaseAngle=Theta_vsc0  Voltage_phases=[25e3 25e3 25e3]/sqrt(3)  PhaseAngles_phases=[0 -120 +120]  Frequency=fb  NonIdealSource=off  SpecifyImpedance=off  Resistance=0  Inductance=0  ShortCircuitLevel=100e6  BaseVoltage=VSC01_Un1  XRratio=7  BusType=swing  Pref=0.3  Qref=0  Prefabc=[10e3, 10e3, 10e3]  Qrefabc=[0, 0, 0]  Qmin=-Inf  Qmax=Inf
  Universal Bridge : powerlib/Power Electronics/Universal Bridge  Arms=3  SnubberResistance=1e5  SnubberCapacitance=inf  Device=Average-model based VSC  Ron=1e-3  Lon=0  ForwardVoltages="[  0  0  ]"  ForwardVoltage=0  GTOparameters=[ 10e-6 , 20e-6 ]  IGBTparameters=[ 1e-6 , 2e-6 ]  Measurements=None  Measurements_2=None  converterType=Rectifier
  Vdc : powerlib/Measurements/Voltage Measurement  PhasorSimulation=off  OutputType=Complex  PSBequivalent=0
  mp3 : Gain  Gain=2/Udcn
  PhA : PMIOPort  Side=Right
  PhB : PMIOPort  Port=2  Side=Right
  PhC : PMIOPort  Port=3  Side=Right
  Vdc+ : PMIOPort  Port=4  Side=Left
  Vdc- : PMIOPort  Port=5  Side=Left
  wires:
  Vdc/1 -> Terminator/1
  Uref/1 -> mp3/1
  mp3/1 -> Saturation/1
  Constant/1 -> Memory1/1
  NOT1/1 -> Three-Phase Breaker3/1
  Saturation/1 -> Universal Bridge/1
  Memory1/1 -> Three-Phase Breaker2/1, NOT1/1
  connections:
  Vdc-/RConn1 -- Universal Bridge/RConn2 -- Vdc/LConn2
  Vdc+/RConn1 -- Universal Bridge/RConn1 -- Vdc/LConn1
  PhC/RConn1 -- Three-Phase Breaker3/LConn3 -- Three-Phase Breaker2/LConn3
  PhB/RConn1 -- Three-Phase Breaker3/LConn2 -- Three-Phase Breaker2/LConn2
  PhA/RConn1 -- Three-Phase Breaker3/LConn1 -- Three-Phase Breaker2/LConn1
  Three-Phase Breaker2/RConn3 -- Universal Bridge/LConn3
  Three-Phase Breaker2/RConn2 -- Universal Bridge/LConn2
  Three-Phase Breaker2/RConn1 -- Universal Bridge/LConn1
  Three-Phase Breaker3/RConn1 -- Three-Phase Source/RConn1
  Three-Phase Breaker3/RConn2 -- Three-Phase Source/RConn2
  Three-Phase Breaker3/RConn3 -- Three-Phase Source/RConn3
